simulink model "EncodersDistancia"  (R2023b)
settings: Solver=FixedStepDiscrete  StartTime=0.0  StopTime=inf  FixedStep=0.01  RelTol=1e-3  EnableMultiTasking=on
libraries: arduinolib x6, arduinosensorlib x2, simulink x2
settings Model: ExtModeTrigDuration=2  Creator=pcele  LastModifiedBy=pcele
settings OptimizationCC: EnhancedBackFolding=on  PassReuseOutputArgsAs=Individual arguments  ZeroExternalMemoryAtStartup=off  ZeroInternalMemoryAtStartup=off  MaxStackSize=64  OptimizeBlockOrder=speed  DifferentSizesBufferReuse=on  OptimizationCustomize=off  EfficientTunableParamExpr=on
settings DebuggingCC: ParameterTunabilityLossMsg=error
settings HardwareCC: ProdBitPerInt=16  ProdBitPerPointer=16  ProdBitPerSizeT=16  ProdBitPerPtrDiffT=16  ProdLargestAtomicFloat=None  ProdWordSize=8  ProdHWDeviceType=Atmel->AVR
settings SFSimCC: MATLABDynamicMemAlloc=off
settings RTWCC: Description=Embedded Coder  SystemTargetFile=ert.tlc  HardwareBoard=Arduino Mega 2560  TemplateMakefile=ert_default_tmf  Toolchain=Arduino AVR  BuildConfiguration=Faster Runs
settings CodeAppCC: ForceParamTrailComments=on  IgnoreCustomStorageClasses=off  OperatorAnnotations=on  SimulinkDataObjDesc=on  SFDataObjDesc=on  InsertBlockDesc=on
settings ERTTargetCC: SupportContinuousTime=on  SupportVariableSizeSignals=on  ExtModeTransport=3  ExtModeStaticAlloc=on  ExtModeAutomaticAllocSize=off  ExtModeStaticAllocSize=2048  ExtModeMexFile=ext_xcp  ExtModeIntrfLevel=Level2 - Open

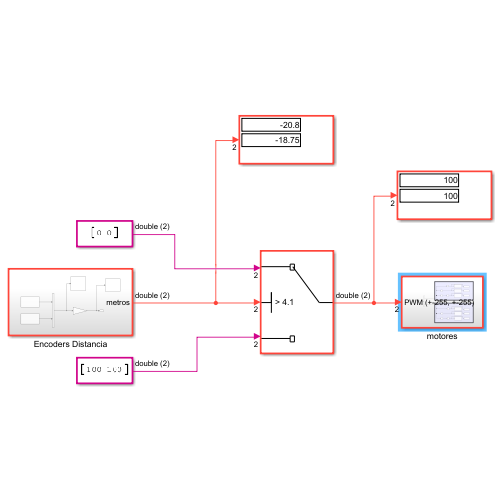
[thumbnail: Simulink's stored preview of the top-level diagram]
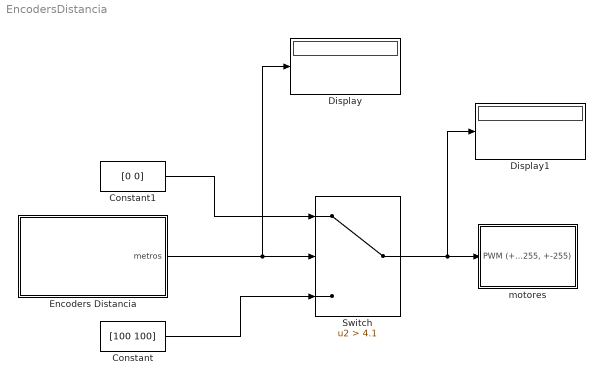
== system EncodersDistancia ==
  Constant : Constant  Value=[100 100]
  Constant1 : Constant  Value=[0 0]
  Display : Display
  Display1 : Display
  Encoders Distancia : Subsystem
  Switch : Switch  Criteria=u2 > Threshold  Threshold=4.1  SaturateOnIntegerOverflow=off  InputSameDT=off
  motores : Subsystem
  wires:
  Encoders Distancia/1(metros) -> Display/1, Switch/2
  Switch/1 -> Display1/1, motores/1("PWM (+-255, +-255)")
  Constant/1 -> Switch/3
  Constant1/1 -> Switch/1

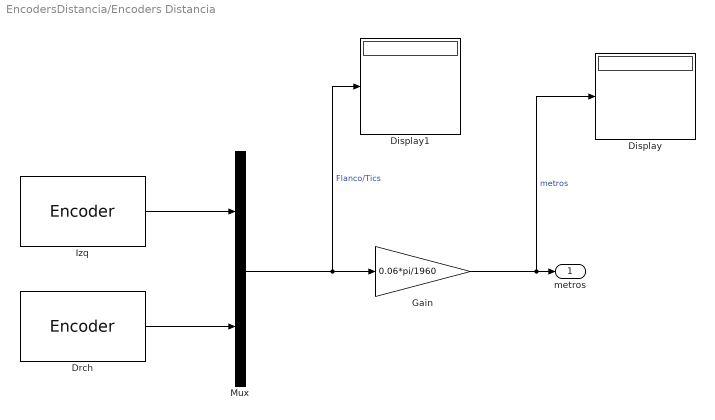
== system EncodersDistancia/Encoders Distancia ==
  Display : Display
  Display1 : Display
  Drch : arduinosensorlib/Encoder  InputA=2  InputB=3  Mode=No reset  SampleTime=-1
  Gain : Gain  Gain=0.06*pi/1960  ParamDataTypeStr=double
  Izq : arduinosensorlib/Encoder  InputA=18  InputB=19  Mode=No reset  SampleTime=-1
  Mux : Mux  Inputs=2
  metros : Outport
  wires:
  Gain/1 -> Display/1, metros/1  "metros"
  Mux/1 -> Display1/1, Gain/1  "Flanco/Tics"
  Drch/1 -> Mux/2
  Izq/1 -> Mux/1

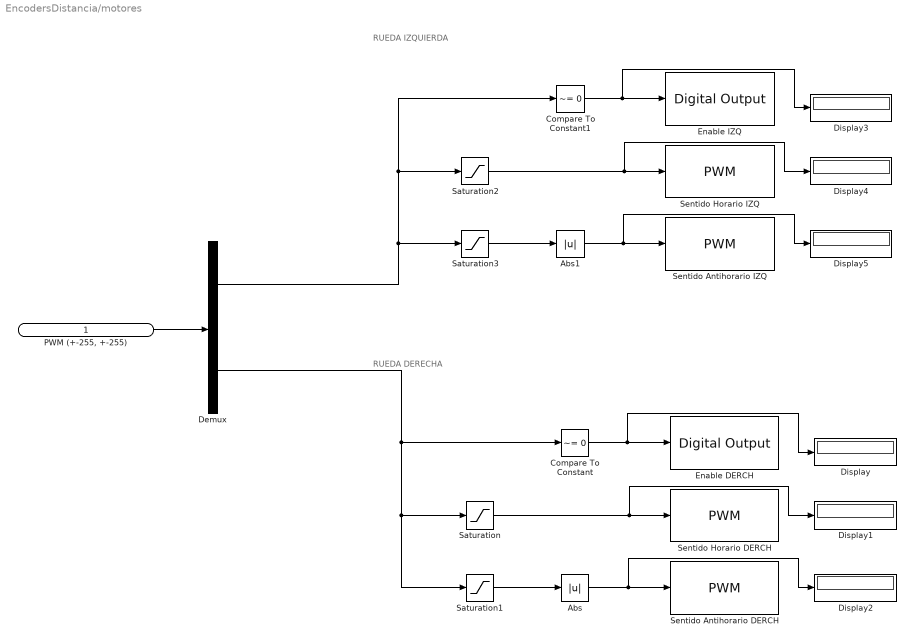
== system EncodersDistancia/motores ==
  note: RUEDA IZQUIERDA
  note: RUEDA DERECHA
  "PWM (+-255, +-255)" : Inport
  Abs : Abs  SaturateOnIntegerOverflow=off
  Abs1 : Abs  SaturateOnIntegerOverflow=off
  Compare To Constant : simulink/Logic and Bit Operations/Compare To Constant  relop=~=  const=0  OutDataTypeStr=boolean
  Compare To Constant1 : simulink/Logic and Bit Operations/Compare To Constant  relop=~=  const=0  OutDataTypeStr=boolean
  Demux : Demux  Outputs=2
  Display{,1..5} (6 alike) : Display
  Enable DERCH : arduinolib/Digital Output  pinNumber=13  Direction=output  blockPlatform=arduino
  Enable IZQ : arduinolib/Digital Output  pinNumber=8  Direction=output  blockPlatform=arduino
  Saturation : Saturate  UpperLimit=255  LowerLimit=0
  Saturation1 : Saturate  UpperLimit=0  LowerLimit=-255
  Saturation2 : Saturate  UpperLimit=255  LowerLimit=0
  Saturation3 : Saturate  UpperLimit=0  LowerLimit=-255
  Sentido Antihorario DERCH : arduinolib/PWM  pinNumber=12  frequencyType=Default  desiredFrequency=490.2  achievableFrequency=490.2
  Sentido Antihorario IZQ : arduinolib/PWM  pinNumber=10  frequencyType=Default  desiredFrequency=490.2  achievableFrequency=490.2
  Sentido Horario DERCH : arduinolib/PWM  pinNumber=11  frequencyType=Default  desiredFrequency=490.2  achievableFrequency=490.2
  Sentido Horario IZQ : arduinolib/PWM  pinNumber=9  frequencyType=Default  desiredFrequency=490.2  achievableFrequency=490.2
  wires:
  Saturation3/1 -> Abs1/1
  Abs/1 -> Display2/1, Sentido Antihorario DERCH/1
  Demux/2 -> Saturation1/1, Saturation/1, Compare To Constant/1
  Abs1/1 -> Display5/1, Sentido Antihorario IZQ/1
  Compare To Constant1/1 -> Display3/1, Enable IZQ/1
  Demux/1 -> Compare To Constant1/1, Saturation2/1, Saturation3/1
  Saturation2/1 -> Sentido Horario IZQ/1, Display4/1
  Saturation/1 -> Sentido Horario DERCH/1, Display1/1
  Compare To Constant/1 -> Display/1, Enable DERCH/1
  Saturation1/1 -> Abs/1
  "PWM (+-255, +-255)"/1 -> Demux/1
